simulink model "solar_cell_simscape"  (R2014a)
settings: Solver=ode23t  StartTime=0.0  StopTime=20  FixedStep=5e-5  RelTol=1e-5
values from neighbouring files (symbols this model uses):
  ArrayCurrent = [1.05303e-05 0.0329007487024 0.0659314357778 0.100205 0.132978217474 0.166891516648 0.200872978445 0.234107600227 0.267513340222 0.302009988541 0.336322 0.36979130469 ... (44440 elements, 101x440)]    [ArrayCurrent.mat]    (also in Genrate_SC_mod.m = fitresult_normal_g42(V,G); temp3.m = fitresult(V,G))
  ArrayVoltage = [0 0.01 0.02 0.03 0.04 0.05 0.06 0.07 0.08 0.09 0.1 0.11 ... (440 elements, 1x440)]    [ArrayVoltage.mat]    (also in Genrate_SC_mod.m = (0:0.01:max(Voltage)); temp3.m = (0:0.01:max(Voltage)))
  Irradiance = (min(Lux):50:max(Lux))    [Genrate_SC_mod.m]    (also in Irradiance.mat = [0 50 100 150 200 250 300 350 400 450 500 550 ... (101 eleme; temp3.m)
libraries: fl_lib x13, nesl_utility x8, simulink x2, elec_lib x2, simulink_extras x1
settings Model: Creator=kartik.karuna  LastModifiedBy=kartik.karuna
settings DebuggingCC: MaxConsecutiveZCsMsg=none

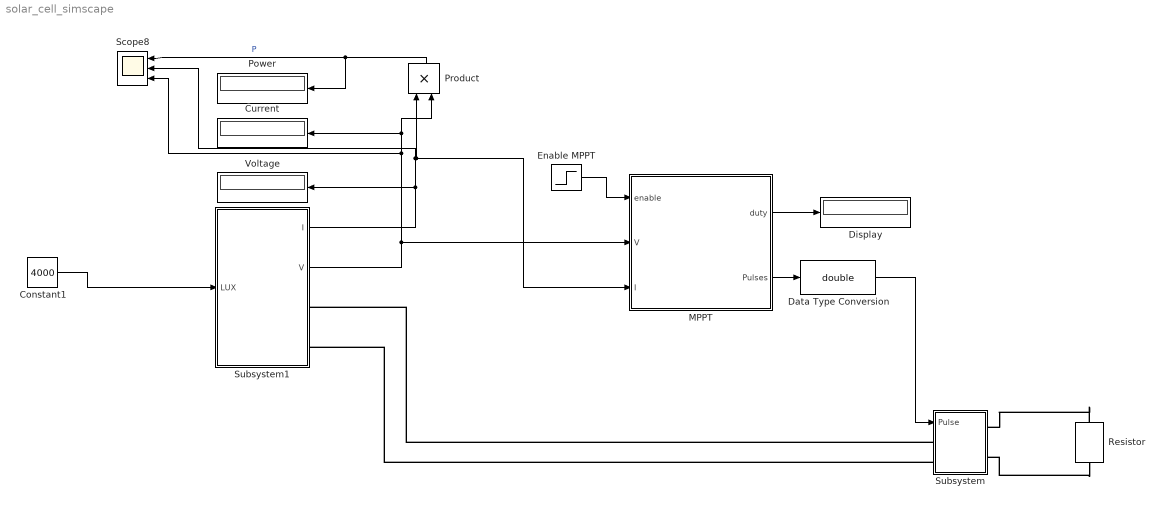
== system solar_cell_simscape ==
  Constant1 : Constant  Value=4000
  Current : Display
  Data Type Conversion : DataTypeConversion  OutDataTypeStr=double
  Display : Display
  Enable MPPT : Step  Time=0.002  SampleTime=0
  MPPT : Subsystem  Variant=on
  Power : Display
  Product : Product  RndMeth=Zero
  Resistor : fl_lib/Electrical/Electrical Elements/Resistor  R=30 Ohm  i_specify=off  i_priority=High  i=0 A  v_specify=off  v_priority=High  v=0 V
  Scope8 : Scope  NumInputPorts=3
      settings: YMin=-1e+07~2~-4e+06  YMax=2e+07~2.75~7e+06  SaveName=ScopeData9
  Subsystem : Subsystem
  Subsystem1 : Subsystem
  Voltage : Display
  wires:
  Enable MPPT/1 -> MPPT/1(enable)
  Product/1 -> Scope8/1, Power/1  "P"
  MPPT/2(Pulses) -> Data Type Conversion/1
  Data Type Conversion/1 -> Subsystem/1(Pulse)
  MPPT/1(duty) -> Display/1
  Subsystem1/2(V) -> Scope8/3, Product/2, Current/1, MPPT/2(V)
  Subsystem1/1(I) -> Scope8/2, Product/1, MPPT/3(I), Voltage/1
  Constant1/1 -> Subsystem1/1(LUX)
  connections:
  Resistor/LConn1 -- Subsystem/RConn1
  Resistor/RConn1 -- Subsystem/RConn2
  Subsystem/LConn1 -- Subsystem1/RConn1
  Subsystem/LConn2 -- Subsystem1/RConn2

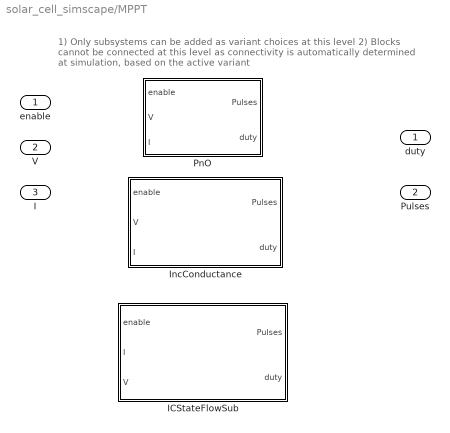
== system solar_cell_simscape/MPPT ==
  note: 1) Only subsystems can be added as variant choices at this level
      | 2) Blocks cannot be connected at this level as connectivity is
      | automatically determined at simulation, based on the active variant
  enable : Inport
  V : Inport  Port=2
  I : Inport  Port=3
  ICStateFlowSub : Subsystem  VariantControl=MPPT_IC_SF
  IncConductance : Subsystem  VariantControl=MPPT_IC_logic
  PnO : Subsystem  VariantControl=MPPT_PnO
  duty : Outport
  Pulses : Outport  Port=2

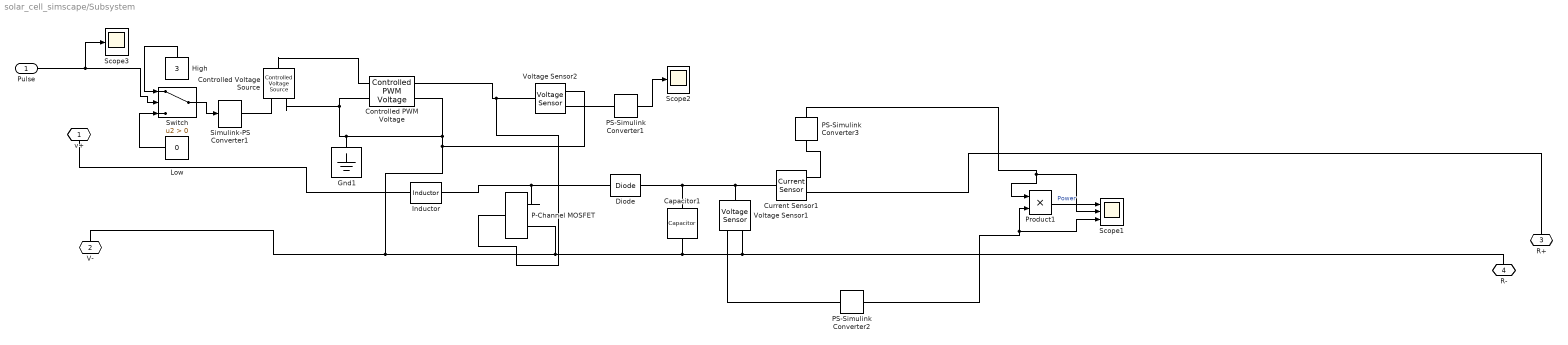
== system solar_cell_simscape/Subsystem ==
  Pulse : Inport
  Capacitor1 : fl_lib/Electrical/Electrical Elements/Capacitor  c=33e-6 F  r=1e-6 Ohm  g=0 1/Ohm  i_specify=off  i_priority=High  i=0 A  v_specify=off  v_priority=High  v=0 V  vc_specify=off  vc_priority=High  vc=0 V
  Controlled PWM Voltage : elec_lib/Actuators & Drivers/Drivers/Controlled PWM Voltage  F=1 Hz  TD=0 s  pulse_width_offset=0 s  Vmin=0 V  Vmax=3 V  Vm=3 V  pwm_or_av=1  event_type=1  sample_time=1e-6 s
  Controlled Voltage Source : fl_lib/Electrical/Electrical Sources/Controlled Voltage Source
  Current Sensor1 : fl_lib/Electrical/Electrical Sensors/Current Sensor
  Diode : fl_lib/Electrical/Electrical Elements/Diode  Vf=0.6 V  Ron=1e-4 Ohm  Goff=1e-8 1/Ohm  i_specify=off  i_priority=High  i=0 A  v_specify=off  v_priority=High  v=0 V
  Gnd1 : fl_lib/Electrical/Electrical Elements/Electrical Reference
  High : Constant  Value=3
  Inductor : fl_lib/Electrical/Electrical Elements/Inductor  l=5e-3 H  r=0.005 Ohm  g=1e-9 1/Ohm  i_specify=off  i_priority=High  i=0 A  v_specify=off  v_priority=High  v=0 V  i_L_specify=off  i_L_priority=High  i_L=0 A
  Low : Constant  Value=0
  P-Channel MOSFET : elec_lib/Semiconductor Devices/P-Channel MOSFET  parameterization=1  prmDatasheet=1  prmEquCoeff=1  Beta=2 A/V^2  Rds=0.167 Ohm  Id=-2.5 A  Vgs=-4.5 V  Vth=-1.4 V  lam=0 1/V  Tmeas=25 C  RS=1e-4 Ohm  RD=0.01 Ohm  C_param=1  C_GS=225 pF  C_GD=45 pF  C_iss=270 pF  C_rss=45 pF  C_oss=0 pF  charge_linearity_param=1  C_OX=200 pF  V_C_OX=0.5 V  dVth_dT=2 mV/K  Rds_T2=0.25 Ohm  Tmeas2=125 C  BEXDatasheet=-1.5  BEXEquCoeff=-1.5  TdeviceDatasheet=25 C  TdeviceEquCoeff=25 C  Rth=[ 0 10 ] K/W  thermal_mass_parameterization=1  thermal_mass=[ 0 1 ] J/K  thermal_time_constant=[ 0 10 ] s  thermal_mass_initial_temperatures=[ 25 25 ] C
  PS-Simulink Converter1 : nesl_utility/PS-Simulink Converter  PhysicalDomain=network_engine_domain  SubClassName=ps_output  LeftPortType=input  RightPortType=output  PseudoPeriodic=off  Frequencies=[]  Unit=1  AffineConversion=off
  PS-Simulink Converter2 : nesl_utility/PS-Simulink Converter  PhysicalDomain=network_engine_domain  SubClassName=ps_output  LeftPortType=input  RightPortType=output  PseudoPeriodic=off  Frequencies=[]  Unit=1  AffineConversion=off
  PS-Simulink Converter3 : nesl_utility/PS-Simulink Converter  PhysicalDomain=network_engine_domain  SubClassName=ps_output  LeftPortType=input  RightPortType=output  PseudoPeriodic=off  Frequencies=[]  Unit=1  AffineConversion=off
  Product1 : Product  RndMeth=Zero
  Scope1 : Scope  NumInputPorts=3
      settings: YMin=0.86~0.1695~5.085  YMax=0.8925~0.1725~5.17
  Scope2 : Scope
      settings: YMin=3  YMax=3
  Scope3 : Scope
      settings: YMin=0.95  YMax=1.05  SaveName=ScopeData2
  Simulink-PS Converter1 : nesl_utility/Simulink-PS Converter  PhysicalDomain=network_engine_domain  SubClassName=ps_input  LeftPortType=input  RightPortType=output  PseudoPeriodic=off  Frequencies=[]  NoiseDistribution=none  NoiseParameters=[]  Unit=1  AffineConversion=off  InputFiltering=off  SimscapeFilterOrder=1  InputFilterTimeConstant=0.001  UdotUserProvided=1
  Switch : Switch  Criteria=u2 > Threshold
  Voltage Sensor1 : fl_lib/Electrical/Electrical Sensors/Voltage Sensor
  Voltage Sensor2 : fl_lib/Electrical/Electrical Sensors/Voltage Sensor
  v+ : PMIOPort  Port=1  Side=Left
  V- : PMIOPort  Port=2  Side=Left
  R+ : PMIOPort  Port=3  Side=Right
  R- : PMIOPort  Port=4  Side=Right
  wires:
  PS-Simulink Converter2/1 -> Scope1/3, Product1/2
  PS-Simulink Converter3/1 -> Scope1/2, Product1/1
  Switch/1 -> Simulink-PS Converter1/1
  Low/1 -> Switch/3
  High/1 -> Switch/1
  Pulse/1 -> Scope3/1, Switch/2
  PS-Simulink Converter1/1 -> Scope2/1
  Product1/1 -> Scope1/1  "Power"
  connections:
  R+/RConn1 -- Current Sensor1/RConn2
  Current Sensor1/RConn1 -- PS-Simulink Converter3/LConn1
  Controlled PWM Voltage/LConn2 -- Gnd1/LConn1 -- Controlled PWM Voltage/RConn2 -- Voltage Sensor2/RConn2 -- P-Channel MOSFET/RConn2 -- Capacitor1/RConn1 -- R-/RConn1 -- Voltage Sensor1/RConn2 -- V-/RConn1 -- Controlled Voltage Source/RConn2
  Diode/LConn1 -- P-Channel MOSFET/RConn1 -- Inductor/RConn1
  Voltage Sensor1/LConn1 -- Capacitor1/LConn1 -- Diode/RConn1 -- Current Sensor1/LConn1
  PS-Simulink Converter2/LConn1 -- Voltage Sensor1/RConn1
  Inductor/LConn1 -- v+/RConn1
  Controlled PWM Voltage/RConn1 -- P-Channel MOSFET/LConn1 -- Voltage Sensor2/LConn1
  Controlled Voltage Source/LConn1 -- Controlled PWM Voltage/LConn1
  Simulink-PS Converter1/RConn1 -- Controlled Voltage Source/RConn1
  Voltage Sensor2/RConn1 -- PS-Simulink Converter1/LConn1

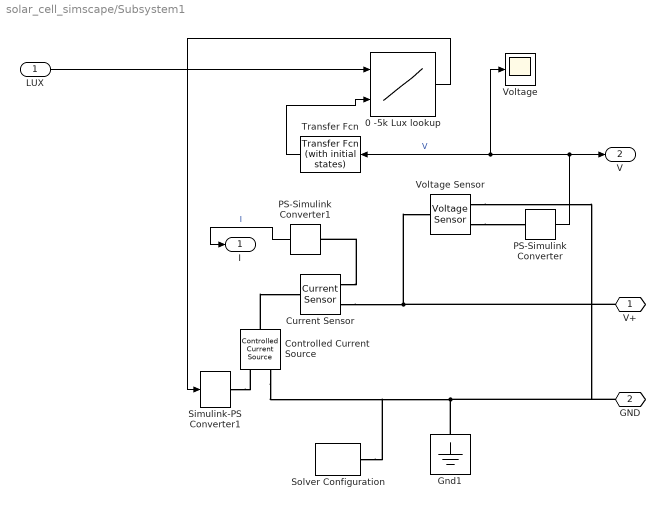
== system solar_cell_simscape/Subsystem1 ==
  LUX : Inport
  0 -5k Lux lookup : Lookup_n-D  BreakpointsForDimension1=Irradiance  BreakpointsForDimension2=ArrayVoltage  Table=ArrayCurrent  RndMeth=Simplest  InputSameDT=on
  Controlled Current Source : fl_lib/Electrical/Electrical Sources/Controlled Current Source
  Current Sensor : fl_lib/Electrical/Electrical Sensors/Current Sensor
  Gnd1 : fl_lib/Electrical/Electrical Elements/Electrical Reference
  PS-Simulink Converter : nesl_utility/PS-Simulink Converter  PhysicalDomain=network_engine_domain  SubClassName=ps_output  LeftPortType=input  RightPortType=output  PseudoPeriodic=off  Frequencies=[]  Unit=1  AffineConversion=off
  PS-Simulink Converter1 : nesl_utility/PS-Simulink Converter  PhysicalDomain=network_engine_domain  SubClassName=ps_output  LeftPortType=input  RightPortType=output  PseudoPeriodic=off  Frequencies=[]  Unit=1  AffineConversion=off
  Simulink-PS Converter1 : nesl_utility/Simulink-PS Converter  PhysicalDomain=network_engine_domain  SubClassName=ps_input  LeftPortType=input  RightPortType=output  PseudoPeriodic=off  Frequencies=[]  NoiseDistribution=none  NoiseParameters=[]  Unit=1  AffineConversion=off  InputFiltering=off  SimscapeFilterOrder=1  InputFilterTimeConstant=0.001  UdotUserProvided=1
  Solver Configuration : nesl_utility/Solver Configuration  PhysicalDomain=network_engine_domain  SubClassName=solver  LeftPortType=input  RightPortType=generic  Accelerate=off  Tones=[]  Harmonics=[]  SimulateNoise=off  Profile=off  UseLocalSampling=off  EnableSwitchedLinearOptims=on  FrequencyDomain=off  UseCCode=off  RelTol=0.001  AbsTol=1e-06  MinStep=1e-09  ToWorkspace=off  DoDC=off  ResidualTolerance=1e-09  UseLocalSolver=off  LocalSolverChoice=NE_BACKWARD_EULER_ADVANCER  LocalSolverSampleTime=0.001  DoFixedCost=off  MaxNonlinIter=3  MaxModeIter=2  LinearAlgebra=Sparse  DelaysMemoryBudget=1024  AutomaticFiltering=on  FilteringTimeConstant=0.001
  Transfer Fcn : simulink_extras/Additional Linear/Transfer Fcn (with initial states)  N=[1]  D="[.0001  1]"  X0=0
  Voltage : Scope
      settings: YMin=0.815936  YMax=0.815936  SaveName=ScopeData6
  Voltage Sensor : fl_lib/Electrical/Electrical Sensors/Voltage Sensor
  V+ : PMIOPort  Port=1  Side=Right
  GND : PMIOPort  Port=2  Side=Right
  I : Outport
  V : Outport  Port=2
  wires:
  0 -5k Lux lookup/1 -> Simulink-PS Converter1/1
  LUX/1 -> 0 -5k Lux lookup/1
  Transfer Fcn/1 -> 0 -5k Lux lookup/2
  PS-Simulink Converter/1 -> V/1, Transfer Fcn/1, Voltage/1  "V"
  PS-Simulink Converter1/1 -> I/1  "I"
  connections:
  Voltage Sensor/RConn1 -- PS-Simulink Converter/LConn1
  Current Sensor/RConn1 -- PS-Simulink Converter1/LConn1
  Controlled Current Source/LConn1 -- Current Sensor/LConn1
  Simulink-PS Converter1/RConn1 -- Controlled Current Source/RConn1
  Current Sensor/RConn2 -- V+/RConn1 -- Voltage Sensor/LConn1
  Gnd1/LConn1 -- Controlled Current Source/RConn2 -- Solver Configuration/RConn1 -- GND/RConn1 -- Voltage Sensor/RConn2

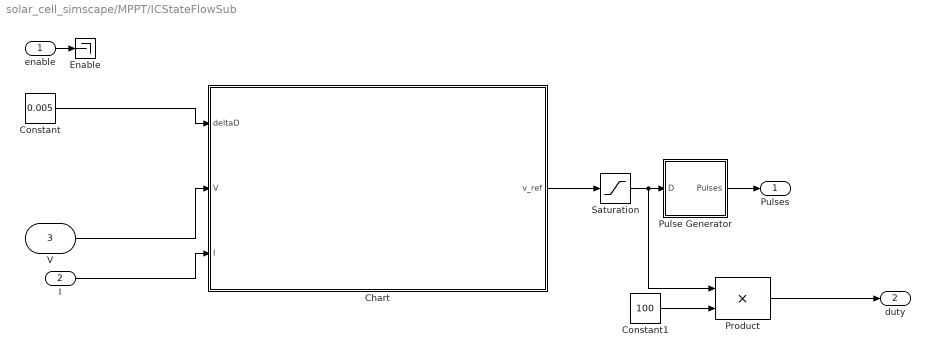
== system solar_cell_simscape/MPPT/ICStateFlowSub ==
  enable : Inport
  I : Inport  Port=2
  V : Inport  Port=3
  Chart : Stateflow chart  TreatAsAtomicUnit=on
  Constant : Constant  Value=0.005
  Constant1 : Constant  Value=100
  "Enable " : Terminator
  Product : Product  RndMeth=Zero
  Pulse Generator : Subsystem  mask{Freq=5000}
      mask prompts: Freq "Frequency (Hz)"
  Saturation : Saturate  UpperLimit=1  LowerLimit=0
  Pulses : Outport
  duty : Outport  Port=2
  wires:
  I/1 -> Chart/3(I)
  Constant/1 -> Chart/1(deltaD)
  V/1 -> Chart/2(V)
  enable/1 -> "Enable "/1
  Chart/1(v_ref) -> Saturation/1
  Pulse Generator/1(Pulses) -> Pulses/1
  Saturation/1 -> Product/1, Pulse Generator/1(D)
  Constant1/1 -> Product/2
  Product/1 -> duty/1

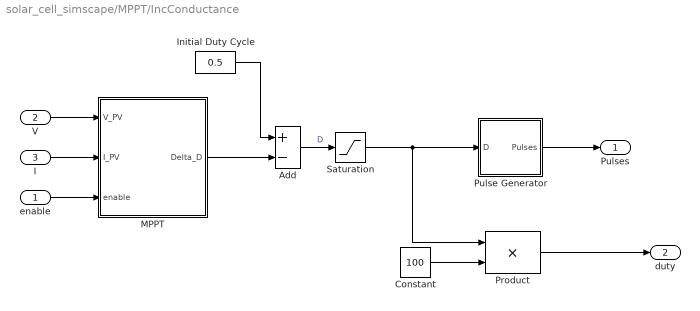
== system solar_cell_simscape/MPPT/IncConductance ==
  enable : Inport
  V : Inport  Port=2
  I : Inport  Port=3
  Add : Sum  Inputs=+-
  Constant : Constant  Value=100
  Initial Duty Cycle : Constant  Value=0.5
  MPPT : Subsystem
  Product : Product  RndMeth=Zero
  Pulse Generator : Subsystem  mask{Freq=5000}
      mask prompts: Freq "Frequency (Hz)"
  Saturation : Saturate  UpperLimit=1  LowerLimit=0  ZeroCross=off
  Pulses : Outport
  duty : Outport  Port=2
  wires:
  Pulse Generator/1(Pulses) -> Pulses/1
  V/1 -> MPPT/1(V_PV)
  Add/1 -> Saturation/1  "D"
  enable/1 -> MPPT/3(enable)
  Initial Duty Cycle/1 -> Add/1
  I/1 -> MPPT/2(I_PV)
  MPPT/1(Delta_D) -> Add/2
  Saturation/1 -> Product/1, Pulse Generator/1(D)
  Constant/1 -> Product/2
  Product/1 -> duty/1

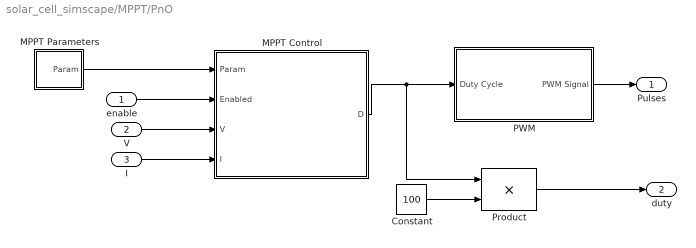
== system solar_cell_simscape/MPPT/PnO ==
  enable : Inport
  V : Inport  Port=2
  I : Inport  Port=3
  Constant : Constant  Value=100
  MPPT Parameters : Subsystem
  "MPPT Control " : MATLAB Function  TreatAsAtomicUnit=on
  PWM : Subsystem  mask(PWM Generator for non bridge applications){fs=50000, A=1}
      mask prompts: fs "Frequency"; A "Amplitude"
      mask help:
      | By default it outputs a 1 unit square wave at 1 hz
      | You can set the duty cycle or use an external line to ajust it on the fly.
  Product : Product  RndMeth=Zero
  Pulses : Outport
  duty : Outport  Port=2
  wires:
  MPPT Parameters/1(Param) -> "MPPT Control "/1(Param)
  enable/1 -> "MPPT Control "/2(Enabled)
  V/1 -> "MPPT Control "/3(V)
  I/1 -> "MPPT Control "/4(I)
  "MPPT Control "/1(D) -> Product/1, PWM/1(Duty Cycle)
  Constant/1 -> Product/2
  Product/1 -> duty/1
  PWM/1(PWM Signal) -> Pulses/1

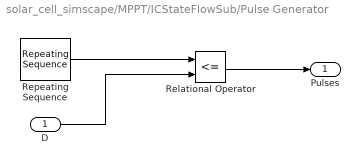
== system solar_cell_simscape/MPPT/ICStateFlowSub/Pulse Generator ==
  D : Inport
  Relational Operator : RelationalOperator  Operator=<=  OutDataTypeStr=boolean
  Repeating Sequence : simulink/Sources/Repeating Sequence  rep_seq_t="[0  1/Freq]"  rep_seq_y=[0 1]
  Pulses : Outport
  wires:
  Repeating Sequence/1 -> Relational Operator/1
  Relational Operator/1 -> Pulses/1
  D/1 -> Relational Operator/2

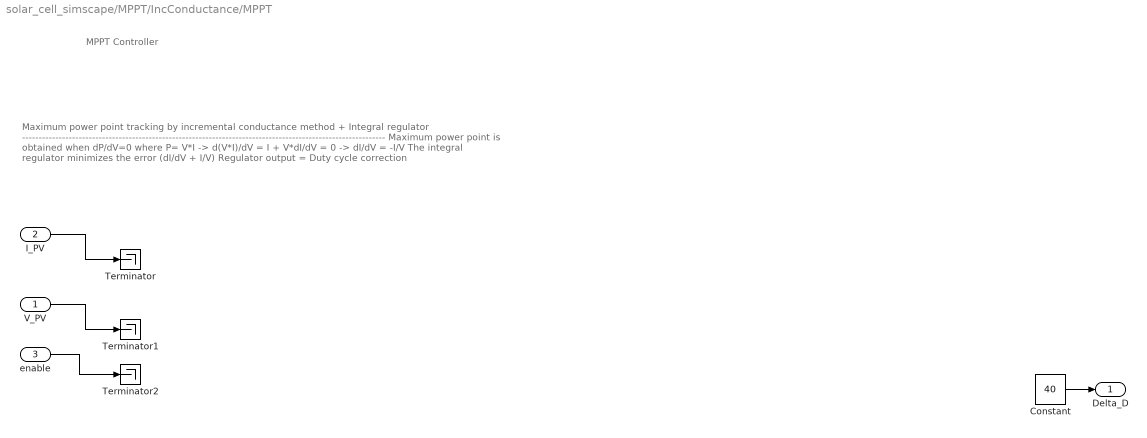
== system solar_cell_simscape/MPPT/IncConductance/MPPT ==
  note: Maximum power point tracking by incremental conductance method + Integral regulator
      | -------------------------------------------------------------------------------------------------------------
      | Maximum power point is obtained when dP/dV=0  where P= V*I
      | -> d(V*I)/dV = I + V*dI/dV = 0
      | -> dI/dV = -I/V
      | The integral regulator minimizes the error (dI/dV + I/V)
      | Regulator output = Duty cycle correction
  note: MPPT Controller
  V_PV : Inport
  I_PV : Inport  Port=2
  enable : Inport  Port=3
  Constant : Constant  Value=40
  Terminator : Terminator
  Terminator1 : Terminator
  Terminator2 : Terminator
  Delta_D : Outport
  wires:
  V_PV/1 -> Terminator1/1
  I_PV/1 -> Terminator/1
  Constant/1 -> Delta_D/1
  enable/1 -> Terminator2/1

== system solar_cell_simscape/MPPT/IncConductance/Pulse Generator ==
  D : Inport
  Relational Operator : RelationalOperator  Operator=<=  OutDataTypeStr=boolean
  Repeating Sequence : simulink/Sources/Repeating Sequence  rep_seq_t="[0  1/Freq]"  rep_seq_y=[0 1]
  Pulses : Outport
  wires:
  D/1 -> Relational Operator/2
  Relational Operator/1 -> Pulses/1
  Repeating Sequence/1 -> Relational Operator/1

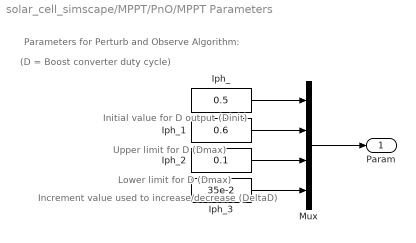
== system solar_cell_simscape/MPPT/PnO/MPPT Parameters ==
  note: Upper limit for D (Dmax)
  note: Increment value used to increase/decrease (DeltaD)
  note: Initial value for D output (Dinit)
  note: (D = Boost converter duty cycle)
  note: Lower limit for D (Dmax)
  note: Parameters for Perturb and Observe Algorithm:
  Iph_ : Constant  Value=0.5
  Iph_1 : Constant  Value=0.6
  Iph_2 : Constant  Value=0.1
  Iph_3 : Constant  Value=35e-2
  Mux : Mux
  Param : Outport
  wires:
  Iph_/1 -> Mux/1
  Iph_1/1 -> Mux/2
  Iph_2/1 -> Mux/3
  Iph_3/1 -> Mux/4
  Mux/1 -> Param/1

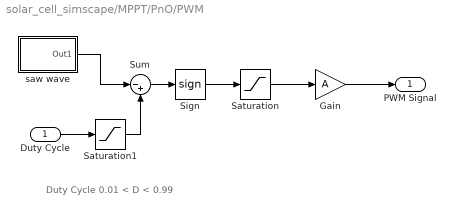
== system solar_cell_simscape/MPPT/PnO/PWM ==
  note: Duty Cycle 0.01 < D < 0.99
  Duty Cycle : Inport
  Gain : Gain  Gain=A
  Saturation : Saturate  UpperLimit=1  LowerLimit=0
  Saturation1 : Saturate  UpperLimit=0.99  LowerLimit=0.01
  Sign : Signum
  Sum : Sum  Inputs=|-+
  saw wave : Subsystem  mask{fs=fs}
      mask init:
      | x=[-1 NaN 4 NaN 0 1 1 2 2 3 3];
      | y=[-0.5 NaN 1.5 NaN 0 1 0 1 0 1 0];
      mask Display:
      | plot(x,y);
      | port_label('output',1,'S')
  PWM Signal : Outport
  wires:
  saw wave/1(Out1) -> Sum/1
  Sum/1 -> Sign/1
  Sign/1 -> Saturation/1
  Saturation/1 -> Gain/1
  Gain/1 -> PWM Signal/1
  Saturation1/1 -> Sum/2
  Duty Cycle/1 -> Saturation1/1

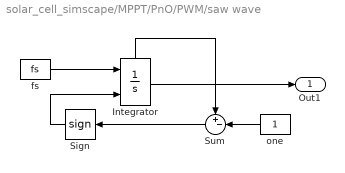
== system solar_cell_simscape/MPPT/PnO/PWM/saw wave ==
  Integrator : Integrator  ExternalReset=rising  ShowStatePort=on
  Sign : Signum
  Sum : Sum  Inputs=+-|
  fs : Constant  Value=fs
  one : Constant
  Out1 : Outport
  wires:
  Integrator/1 -> Out1/1
  Sum/1 -> Sign/1
  fs/1 -> Integrator/1
  one/1 -> Sum/2
  Sign/1 -> Integrator/2
  Integrator/State -> Sum/1

== matlab function solar_cell_simscape/MPPT/PnO/MPPT Control  ==
  settings: updateMethod=DISCRETE  sampleTime=Ts_Control
  data: Param input; Enabled input; V input; I input; D output
function D  = PandO(Param, Enabled, V, I)

% MPPT controller based on the Perturb & Observe algorithm.

% D output = Duty cycle  (value between 0 and 1)
%
% Enabled input = 1 to enable the MPPT controller
% V input = PV array terminal voltage (V)
% I input = PV array current (A)
%
% Param input:
Dinit = Param(1);  %Initial value for D output
Dmax = Param(2);   %Maximum value for D
Dmin = Param(3);   %Minimum value for D
deltaD = Param(4); %Increment value used to increase/decrease the duty cycle D
% ( increasing D = decreasing Vref )


persistent Vold Pold Dold;

dataType = 'double';

if isempty(Vold)
    Vold=0;
    Pold=0;
    Dold=Dinit;
end
P= V*I;
dV= V - Vold;
dP= P - Pold;

if dP ~= 0 & Enabled ~=0
    if dP < 0
        if dV < 0
            D = Dold - deltaD;
        else
            D = Dold + deltaD;
        end
    else
        if dV < 0
            D = Dold + deltaD;
        else
            D = Dold - deltaD;
        end    
    end
else D=Dold;
end

if D >= Dmax | D<= Dmin
    D=Dold;
end

Dold=D;
Vold=V;
Pold=P;

== stateflow chart solar_cell_simscape/MPPT/ICStateFlowSub/Chart ==
  state init
    entry:
    V_prev1=0;
    I_prev1=0;
    V_REF=0;
  state Sample_and_call
    entry:
    deltaV = V -V_prev1;
    deltaI = I - I_prev1;
    v_ref = V_REF;
  state INCREMENT
    entry:
    v_ref =v_ref+deltaD;
  state DECREMENT
    entry:
    v_ref =v_ref-deltaD;
  state RETURN
    entry:
    V_prev1 = V;
    I_prev1 = I ;
    V_REF= v_ref;
  (default) -> init
  init -> Sample_and_call
  RETURN -> Sample_and_call
  Sample_and_call -> (junction 6) [order 1] : [deltaV==0]
  Sample_and_call -> (junction 22) [order 2] : [deltaV~=0]
  (junction 6) -> RETURN [order 2] : [deltaI==0]
  (junction 6) -> (junction 16) [order 1] : [deltaI~=0]
  (junction 22) -> RETURN [order 2] : [deltaI/deltaV == -(I/V)]
  (junction 22) -> (junction 15) [order 1] : [deltaI/deltaV ~= -(I/V)]
  (junction 16) -> DECREMENT [order 2] : [deltaI<=0]
  (junction 16) -> INCREMENT [order 1] : [deltaI>0]
  (junction 15) -> INCREMENT [order 1] : [deltaI/deltaV > -(I/V)]
  (junction 15) -> DECREMENT [order 2] : [deltaI/deltaV <= -(I/V)]
  INCREMENT -> RETURN
  DECREMENT -> RETURN
  data: deltaD input; v_ref output double; V_prev1 local =0; I_prev1 local =0; V_REF local =0; deltaV local; deltaI local; V input; I input
